simulink model "dryclutchexpsim"  (Simulink 5.0)
settings: Solver=ode23  SolverMode=SingleTasking  StartTime=0.0  StopTime=Tstop  RelTol=1e-5  AbsTol=1e-6
values from neighbouring files (symbols this model uses):
  be = 0.03    [init.m]
  bv = 0.03    [init.m]
  E = expcon(C,range)    [explicit.m]    (also in init.m = expcon(C,range,options))
  Ie = 0.2    [init.m]
  Iv = 0.7753    [init.m]
  mud = 0.4    [init.m]
  muk = 1    [init.m]
  mus = 1.5    [init.m]
  R = 3*k/(4*mud)    (= 0.18375)    [init.m]    (also in plotresults.m = 3*k/(4*mud))
  Ts = .01    (= 0.01)    [init.m]
  we0 = 95    [init.m]
  wv0 = 0    [init.m]
libraries: hyblib x1
settings Model: LastModifiedBy=Alberto Bemporad  ExtModeTrigMode=oneshot  ExtModeArmWhenConnect=off  ExternalInput=[]  InitialState=[]  TimeSaveName=t  SaveState=on  StateSaveName=x  OutputSaveName=y  LimitDataPoints=off  IntegerOverflowMsg=none  BooleanDataType=off

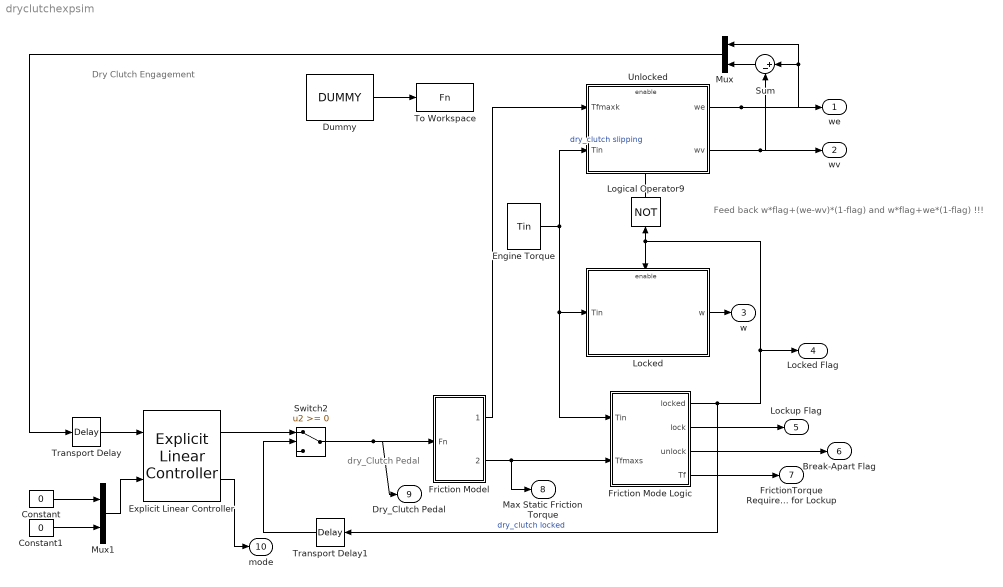
== system dryclutchexpsim ==
  note: Dry Clutch Engagement
  note: dry_Clutch
      | Pedal
  note: Feed back w*flag+(we-wv)*(1-flag)
      | and   w*flag+we*(1-flag)   !!!
  Constant : Constant  Value=0
  Constant1 : Constant  Value=0
  Dummy : FromWorkspace  VariableName=DUMMY  SampleTime=0
  Engine Torque : FromWorkspace  VariableName=Tin  SampleTime=0
  Explicit Linear Controller : hyblib/Explicit Linear Controller  C=E  xhat0=xhat0  u1=u0  compile=on
  Friction Model : Subsystem
  Friction Mode Logic : Subsystem
      mask Display: plot([-3 1 1 3 -1 -1],[-1 -1 1 1 1 -1],-4,-5,4,5)
  Locked : Subsystem
      mask Display: plot(-1,-6,6,12,[0 3],[3 3],[3 1 1 3], [1 1 5 5],[2 4 4 2],[4 4 2 2],[4 5],[3 3])
  Logical Operator9 : Logic  Orientation=up  Operator=NOT  Inputs=1
      mask Display: plot(0, -.25, 2., .5, [0 2 0 0], [-.5 0 .5 -.5],.2*cos(0:.1:2*pi)+2.2, .1*sin(0:.1:2*pi))
  Mux : Mux  Orientation=left  Inputs=2
  Mux1 : Mux  Inputs=2
  Sum : Sum  Orientation=left  Inputs=|+-  SaturateOnIntegerOverflow=on  InputSameDT=on
  Switch2 : Switch  SaturateOnIntegerOverflow=on
  To Workspace : ToWorkspace  VariableName=Fn  SampleTime=-1  SaveFormat=Array
  Transport Delay : TransportDelay  DelayTime=Ts/100
  Transport Delay1 : TransportDelay  Orientation=left  DelayTime=Ts/100
  Unlocked : Subsystem
      mask Display: plot(-1,-2,6,8,[0 3],[3 3],[3 1 1 3], [1 1 5 5],[2 4 4 2],[4 4 2 2],[4 5],[3 3])
  we : Outport  InitialOutput=0
  wv : Outport  Port=2  InitialOutput=0
  w : Outport  Port=3  InitialOutput=0
  Locked Flag : Outport  Port=4  InitialOutput=0
  Lockup Flag : Outport  Port=5  InitialOutput=0
  Break-Apart Flag : Outport  Port=6  InitialOutput=0
  FrictionTorque Required for Lockup : Outport  Port=7  InitialOutput=0
  Max Static Friction Torque : Outport  Port=8  InitialOutput=0
  Dry_Clutch Pedal : Outport  Port=9  InitialOutput=0
  mode : Outport  Port=10  InitialOutput=0
  wires:
  Friction Mode Logic/3(unlock) -> Break-Apart Flag/1
  Engine Torque/1 -> Locked/1(Tin), Friction Mode Logic/1(Tin), Unlocked/2(Tin)
  Friction Model/1(Tfmaxk) -> Unlocked/1(Tfmaxk)
  Friction Mode Logic/2(lock) -> Lockup Flag/1
  Friction Mode Logic/4(Tf) -> FrictionTorque Required for Lockup/1
  Locked/1(w) -> w/1
  Logical Operator9/1 -> Unlocked/Enable  "dry_clutch slipping"
  Friction Model/2(Tfmaxs) -> Friction Mode Logic/2(Tfmaxs), Max Static Friction Torque/1
  Sum/1 -> Mux/2
  Dummy/1 -> To Workspace/1
  Mux/1 -> Transport Delay/1
  Friction Mode Logic/1(locked) -> Locked Flag/1, Logical Operator9/1, Locked/Enable, Transport Delay1/1  "dry_clutch locked"
  Unlocked/1(we) -> we/1, Mux/1, Sum/1
  Unlocked/2(wv) -> wv/1, Sum/2
  Constant/1 -> Mux1/1
  Constant1/1 -> Mux1/2
  Mux1/1 -> Explicit Linear Controller/2
  Transport Delay/1 -> Explicit Linear Controller/1
  Explicit Linear Controller/1 -> Switch2/1
  Switch2/1 -> Friction Model/1(Fn), Dry_Clutch Pedal/1
  Explicit Linear Controller/2 -> mode/1
  Transport Delay1/1 -> Switch2/2

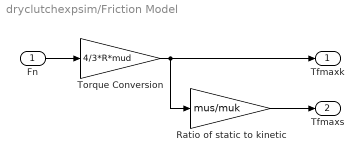
== system dryclutchexpsim/Friction Model ==
  Fn : Inport
  Ratio of static to kinetic : Gain  Gain=mus/muk  SaturateOnIntegerOverflow=on
  Torque Conversion : Gain  Gain=4/3*R*mud  SaturateOnIntegerOverflow=on
  Tfmaxk : Outport  InitialOutput=0
  Tfmaxs : Outport  Port=2  InitialOutput=0
  wires:
  Torque Conversion/1 -> Tfmaxk/1, Ratio of static to kinetic/1
  Fn/1 -> Torque Conversion/1
  Ratio of static to kinetic/1 -> Tfmaxs/1

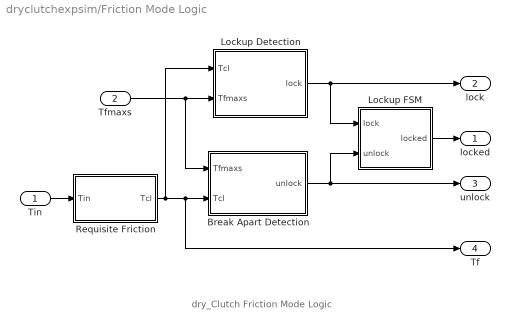
== system dryclutchexpsim/Friction Mode Logic ==
  note: dry_Clutch Friction Mode Logic
  Tin : Inport
  Tfmaxs : Inport  Port=2
  Break Apart Detection : Subsystem
  Lockup Detection : Subsystem
  Lockup FSM : Subsystem
  Requisite Friction : Subsystem
  locked : Outport  InitialOutput=0
  lock : Outport  Port=2  InitialOutput=0
  unlock : Outport  Port=3  InitialOutput=0
  Tf : Outport  Port=4  InitialOutput=0
  wires:
  Tfmaxs/1 -> Lockup Detection/2(Tfmaxs), Break Apart Detection/1(Tfmaxs)
  Break Apart Detection/1(unlock) -> Lockup FSM/2(unlock), unlock/1
  Lockup Detection/1(lock) -> Lockup FSM/1(lock), lock/1
  Lockup FSM/1(locked) -> locked/1
  Tin/1 -> Requisite Friction/1(Tin)
  Requisite Friction/1(Tcl) -> Break Apart Detection/2(Tcl), Tf/1, Lockup Detection/1(Tcl)

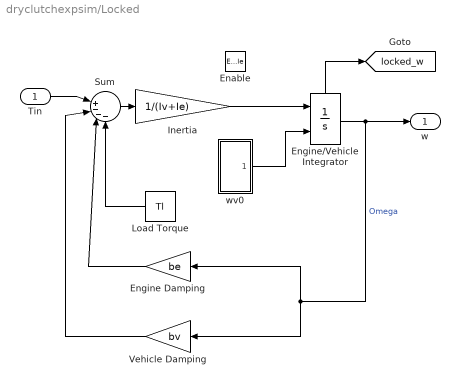
== system dryclutchexpsim/Locked ==
  Tin : Inport
  Enable : EnablePort  StatesWhenEnabling=reset
  Engine Damping : Gain  Orientation=left  Gain=be  SaturateOnIntegerOverflow=on
  Engine/Vehicle Integrator : Integrator  InitialConditionSource=external  ShowStatePort=on
  Inertia : Gain  Gain=1/(Iv+Ie)  SaturateOnIntegerOverflow=on
  Load Torque : FromWorkspace  Orientation=left  VariableName=Tl  SampleTime=0
  Sum : Sum  Inputs=||+---  SaturateOnIntegerOverflow=on  InputSameDT=on
  Vehicle Damping : Gain  Orientation=left  Gain=bv  SaturateOnIntegerOverflow=on
  wv0 : Subsystem
  w : Outport  InitialOutput=0
  tag scope: locked_w=global
  wires:
  Engine/Vehicle Integrator/State -> [locked_w]
  Sum/1 -> Inertia/1
  Tin/1 -> Sum/1
  Engine/Vehicle Integrator/1 -> w/1, Engine Damping/1, Vehicle Damping/1  "Omega"
  Inertia/1 -> Engine/Vehicle Integrator/1
  Engine Damping/1 -> Sum/3
  Vehicle Damping/1 -> Sum/2
  Load Torque/1 -> Sum/4
  wv0/1(Out1) -> Engine/Vehicle Integrator/2

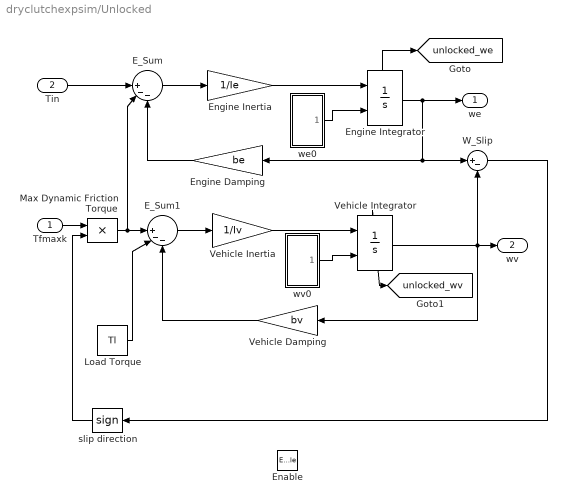
== system dryclutchexpsim/Unlocked ==
  Tfmaxk : Inport
  Tin : Inport  Port=2
  Enable : EnablePort  StatesWhenEnabling=reset
  E_Sum : Sum  Inputs=||+--  SaturateOnIntegerOverflow=on  InputSameDT=on
  E_Sum1 : Sum  Inputs=||+--  SaturateOnIntegerOverflow=on  InputSameDT=on
  Engine Damping : Gain  Orientation=left  Gain=be  SaturateOnIntegerOverflow=on
  Engine Inertia : Gain  Gain=1/Ie  SaturateOnIntegerOverflow=on
  Engine Integrator : Integrator  InitialConditionSource=external  ShowStatePort=on
  Load Torque : FromWorkspace  VariableName=Tl  SampleTime=0
  Max Dynamic Friction Torque : Product  SaturateOnIntegerOverflow=on  InputSameDT=on
  Vehicle Damping : Gain  Orientation=left  Gain=bv  SaturateOnIntegerOverflow=on
  Vehicle Inertia : Gain  Gain=1/Iv  SaturateOnIntegerOverflow=on
  Vehicle Integrator : Integrator  InitialConditionSource=external  ShowStatePort=on
  W_Slip : Sum  Inputs=|+-  SaturateOnIntegerOverflow=on  InputSameDT=on
  slip direction : Signum  Orientation=left
  we0 : Subsystem
  wv0 : Subsystem
  we : Outport  InitialOutput=0
  wv : Outport  Port=2  InitialOutput=0
  tag scope: unlocked_we=global, unlocked_wv=global
  wires:
  E_Sum1/1 -> Vehicle Inertia/1
  Vehicle Damping/1 -> E_Sum1/3
  Max Dynamic Friction Torque/1 -> E_Sum1/1, E_Sum/2
  Tfmaxk/1 -> Max Dynamic Friction Torque/1
  Engine Integrator/State -> [unlocked_we]
  Engine Inertia/1 -> Engine Integrator/1
  E_Sum/1 -> Engine Inertia/1
  Engine Damping/1 -> E_Sum/3
  Engine Integrator/1 -> we/1, Engine Damping/1, W_Slip/1
  Tin/1 -> E_Sum/1
  Vehicle Integrator/State -> [unlocked_wv]
  Vehicle Inertia/1 -> Vehicle Integrator/1
  Vehicle Integrator/1 -> Vehicle Damping/1, wv/1, W_Slip/2
  Load Torque/1 -> E_Sum1/2
  slip direction/1 -> Max Dynamic Friction Torque/2
  W_Slip/1 -> slip direction/1
  we0/1(Out1) -> Engine Integrator/2
  wv0/1(Out1) -> Vehicle Integrator/2

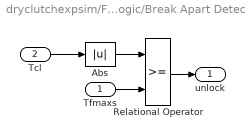
== system dryclutchexpsim/Friction Mode Logic/Break Apart Detection ==
  Tfmaxs : Inport
  Tcl : Inport  Port=2
  Abs : Abs  SaturateOnIntegerOverflow=on
  Relational Operator : RelationalOperator  InputSameDT=on
  unlock : Outport  InitialOutput=0
  wires:
  Tcl/1 -> Abs/1
  Relational Operator/1 -> unlock/1
  Abs/1 -> Relational Operator/1
  Tfmaxs/1 -> Relational Operator/2

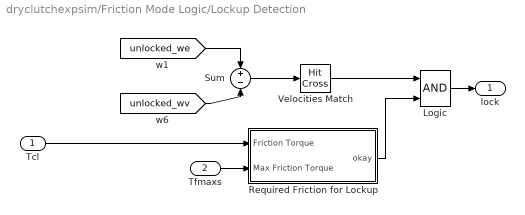
== system dryclutchexpsim/Friction Mode Logic/Lockup Detection ==
  Tcl : Inport
  Tfmaxs : Inport  Port=2
  Logic : Logic
  Required Friction for Lockup : Subsystem
  Sum : Sum  Inputs=+-  SaturateOnIntegerOverflow=on  InputSameDT=on
  Velocities Match : HitCross
  lock : Outport  InitialOutput=0
  wires:
  Tfmaxs/1 -> Required Friction for Lockup/2(Max Friction Torque)
  Velocities Match/1 -> Logic/1
  Logic/1 -> lock/1
  Required Friction for Lockup/1(okay) -> Logic/2
  [unlocked_we] -> Sum/1
  [unlocked_wv] -> Sum/2
  Sum/1 -> Velocities Match/1
  Tcl/1 -> Required Friction for Lockup/1(Friction Torque)

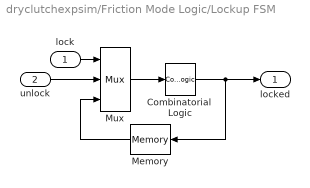
== system dryclutchexpsim/Friction Mode Logic/Lockup FSM ==
  lock : Inport
  unlock : Inport  Port=2
  Combinatorial  Logic : CombinatorialLogic  TruthTable=[0;1;0;0;1;1;1;0]
  Memory : Memory  Orientation=left
  Mux : Mux  Inputs=3
  locked : Outport  InitialOutput=0
  wires:
  Memory/1 -> Mux/3
  Combinatorial  Logic/1 -> locked/1, Memory/1
  unlock/1 -> Mux/2
  lock/1 -> Mux/1
  Mux/1 -> Combinatorial  Logic/1

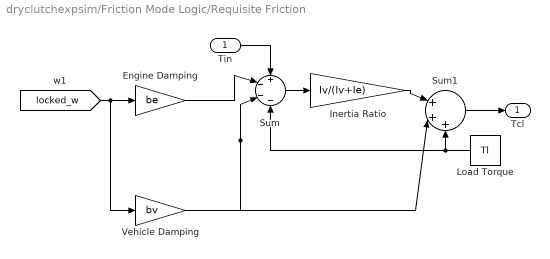
== system dryclutchexpsim/Friction Mode Logic/Requisite Friction ==
  Tin : Inport
  Engine Damping : Gain  Gain=be  SaturateOnIntegerOverflow=on
  Inertia Ratio : Gain  Gain=Iv/(Iv+Ie)  SaturateOnIntegerOverflow=on
  Load Torque : FromWorkspace  Orientation=left  VariableName=Tl  SampleTime=0
  Sum : Sum  Inputs=+---  SaturateOnIntegerOverflow=on  InputSameDT=on
  Sum1 : Sum  Inputs=|+++  SaturateOnIntegerOverflow=on  InputSameDT=on
  Vehicle Damping : Gain  Gain=bv  SaturateOnIntegerOverflow=on
  Tcl : Outport  InitialOutput=0
  wires:
  [locked_w] -> Vehicle Damping/1, Engine Damping/1
  Engine Damping/1 -> Sum/2
  Sum/1 -> Inertia Ratio/1
  Tin/1 -> Sum/1
  Inertia Ratio/1 -> Sum1/1
  Sum1/1 -> Tcl/1
  Vehicle Damping/1 -> Sum/3, Sum1/2
  Load Torque/1 -> Sum/4, Sum1/3

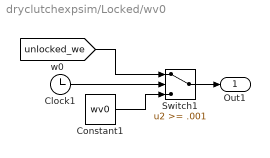
== system dryclutchexpsim/Locked/wv0 ==
  Clock1 : Clock
      settings: Decimation=10
  Constant1 : Constant  Value=wv0
  Switch1 : Switch  Threshold=.001  SaturateOnIntegerOverflow=on  InputSameDT=on
  Out1 : Outport
  wires:
  Clock1/1 -> Switch1/2
  [unlocked_we] -> Switch1/1
  Constant1/1 -> Switch1/3
  Switch1/1 -> Out1/1

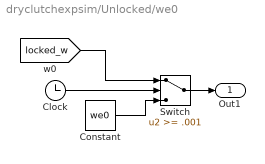
== system dryclutchexpsim/Unlocked/we0 ==
  Clock : Clock
      settings: Decimation=10
  Constant : Constant  Value=we0
  Switch : Switch  Threshold=.001  SaturateOnIntegerOverflow=on  InputSameDT=on
  Out1 : Outport
  wires:
  Clock/1 -> Switch/2
  [locked_w] -> Switch/1
  Constant/1 -> Switch/3
  Switch/1 -> Out1/1

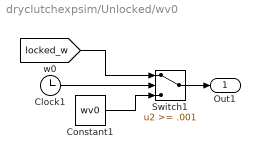
== system dryclutchexpsim/Unlocked/wv0 ==
  Clock1 : Clock
      settings: Decimation=10
  Constant1 : Constant  Value=wv0
  Switch1 : Switch  Threshold=.001  SaturateOnIntegerOverflow=on  InputSameDT=on
  Out1 : Outport
  wires:
  Clock1/1 -> Switch1/2
  [locked_w] -> Switch1/1
  Constant1/1 -> Switch1/3
  Switch1/1 -> Out1/1

== system dryclutchexpsim/Friction Mode Logic/Lockup Detection/Required Friction for Lockup ==
  Friction Torque : Inport
  Max Friction Torque : Inport  Port=2
  Abs : Abs  SaturateOnIntegerOverflow=on
  Relational Operator : RelationalOperator  Operator=<=  InputSameDT=on
  okay : Outport  InitialOutput=0
  wires:
  Friction Torque/1 -> Abs/1
  Relational Operator/1 -> okay/1
  Abs/1 -> Relational Operator/1
  Max Friction Torque/1 -> Relational Operator/2
